simulink library "KR6_Lib"  (R2018a)
settings: Solver=VariableStepAuto  StartTime=0.0  StopTime=10.0  RelTol=1e-3
settings Model: Creator=Pedro Ramalho  LastModifiedBy=Pedro Ramalho

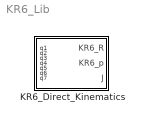
== system KR6_Lib ==
  KR6_Direct_Kinematics : MATLAB Function  TreatAsAtomicUnit=on

== matlab function KR6_Lib/KR6_Direct_Kinematics ==
  data: q1 input; KR6_R output; q2 input; q3 input; q4 input; q5 input; q6 input; q7 input; KR6_p output; J output
function [KR6_R,KR6_p,J] = KR6_Direct_Kinematics(q1,q2,q3,q4,q5,q6,q7)
%#codegen

%    This function was generated by the Symbolic Math Toolbox version 8.1.
%    09-Apr-2020 23:52:27

t2 = cos(q2);
t3 = sin(q2);
t4 = sin(q5);
t5 = cos(q5);
t6 = cos(q3);
t7 = cos(q4);
t8 = sin(q3);
t9 = sin(q4);
t13 = t2.*t6.*t7;
t14 = t2.*t8.*t9;
t10 = t13-t14;
t11 = cos(q7);
t12 = t3.*t5;
t73 = t4.*t10;
t15 = t12-t73;
t16 = sin(q7);
t17 = cos(q6);
t18 = t3.*t4;
t19 = t5.*t10;
t20 = t18+t19;
t21 = sin(q6);
t22 = t2.*t6.*t9;
t23 = t2.*t7.*t8;
t24 = t22+t23;
t25 = t17.*t20-t21.*t24;
t26 = q3+q4;
t27 = sin(t26);
t28 = cos(t26);
t29 = t21.*t28;
t30 = t5.*t17.*t27;
t31 = t29+t30;
t32 = t3.*t6.*t7;
t35 = t3.*t8.*t9;
t33 = t32-t35;
t34 = t2.*t5;
t36 = t4.*t33;
t37 = t34+t36;
t38 = t2.*t4;
t46 = t5.*t33;
t39 = t38-t46;
t40 = t17.*t39;
t41 = t3.*t6.*t9;
t42 = t3.*t7.*t8;
t43 = t41+t42;
t44 = t21.*t43;
t45 = t40+t44;
t47 = t3.*t8.*t9.*(7.0./2.0e2);
t48 = t3.*t17.*t27.*(2.0./2.5e1);
t49 = t3.*t6.*t9.*(7.3e1./2.0e2);
t50 = t3.*t7.*t8.*(7.3e1./2.0e2);
t51 = t3.*t5.*t6.*t7.*t21.*(2.0./2.5e1);
t52 = t28.*(7.3e1./2.0e2);
t53 = t27.*(7.0./2.0e2);
t54 = t8.*(6.3e1./2.0e2);
t55 = q5-q6;
t56 = sin(t55);
t57 = t27.*t56.*(1.0./2.5e1);
t58 = q5+q6;
t59 = sin(t58);
t60 = t17.*t28.*(2.0./2.5e1);
t68 = t27.*t59.*(1.0./2.5e1);
t61 = t52+t53+t54+t57+t60-t68;
t62 = t6.*t7.*(7.0./2.0e2);
t63 = t5.*t8.*t9.*t21.*(2.0./2.5e1);
t64 = t2.*(1.0./4.0e1);
t65 = t2.*t6.*(6.3e1./2.0e2);
t66 = t2.*t6.*t7.*(7.0./2.0e2);
t67 = t2.*t5.*t8.*t9.*t21.*(2.0./2.5e1);
t69 = t28.*7.3e1;
t70 = t27.*7.0;
t71 = t17.*t28.*1.6e1;
t72 = t69+t70+t71-t5.*t21.*t27.*1.6e1;
t74 = t17.*t28;
t75 = t17.*t43;
KR6_R = reshape([t15.*t16+t11.*t25,t11.*t31-t4.*t16.*t27,t16.*t37+t11.*t45,-t11.*t15+t16.*t25,t16.*t31+t4.*t11.*t27,-t11.*t37+t16.*t45,-t17.*t24-t20.*t21,t74-t5.*t21.*t27,t75-t21.*t39],[3,3]);
if nargout > 1
    KR6_p = [t64+t65+t66+t67-t2.*t6.*t9.*(7.3e1./2.0e2)-t2.*t7.*t8.*(7.3e1./2.0e2)-t2.*t8.*t9.*(7.0./2.0e2)-t3.*t4.*t21.*(2.0./2.5e1)-t2.*t17.*t27.*(2.0./2.5e1)-t2.*t5.*t6.*t7.*t21.*(2.0./2.5e1);t61;q1-t3.*(1.0./4.0e1)+t47+t48+t49+t50+t51-t3.*t6.*(6.3e1./2.0e2)-t3.*t6.*t7.*(7.0./2.0e2)-t2.*t4.*t21.*(2.0./2.5e1)-t3.*t5.*t8.*t9.*t21.*(2.0./2.5e1)];
end
if nargout > 2
    J = reshape([0.0,0.0,1.0,0.0,0.0,0.0,t3.*(-1.0./4.0e1)+t47+t48+t49+t50+t51-t3.*t6.*(6.3e1./2.0e2)-t3.*t6.*t7.*(7.0./2.0e2)-t2.*t4.*t21.*(2.0./2.5e1)-t3.*t5.*t8.*t9.*t21.*(2.0./2.5e1),0.0,-t64-t65-t66-t67+t2.*t6.*t9.*(7.3e1./2.0e2)+t2.*t7.*t8.*(7.3e1./2.0e2)+t2.*t8.*t9.*(7.0./2.0e2)+t3.*t4.*t21.*(2.0./2.5e1)+t2.*t17.*t27.*(2.0./2.5e1)+t2.*t5.*t6.*t7.*t21.*(2.0./2.5e1),0.0,1.0,0.0,-t2.*t61,t6.*(6.3e1./2.0e2)+t62+t63-t6.*t9.*(7.3e1./2.0e2)-t7.*t8.*(7.3e1./2.0e2)-t8.*t9.*(7.0./2.0e2)-t6.*t9.*t17.*(2.0./2.5e1)-t7.*t8.*t17.*(2.0./2.5e1)-t5.*t6.*t7.*t21.*(2.0./2.5e1),t3.*t61,t3,0.0,t2,t2.*t72.*(-1.0./2.0e2),t62+t63-t6.*t9.*(7.3e1./2.0e2)-t7.*t8.*(7.3e1./2.0e2)-t8.*t9.*(7.0./2.0e2)-t6.*t9.*t17.*(2.0./2.5e1)-t7.*t8.*t17.*(2.0./2.5e1)-t5.*t6.*t7.*t21.*(2.0./2.5e1),t3.*t72.*(1.0./2.0e2),t3,0.0,t2,t21.*(t12-t2.*t4.*t6.*t7+t2.*t4.*t8.*t9).*(-2.0./2.5e1),t4.*t21.*t27.*(2.0./2.5e1),t21.*(t34+t3.*t4.*t6.*t7-t3.*t4.*t8.*t9).*(-2.0./2.5e1),t2.*t27,-t28,-t3.*t27,t3.*t4.*t17.*(-2.0./2.5e1)+t2.*t6.*t9.*t21.*(2.0./2.5e1)+t2.*t7.*t8.*t21.*(2.0./2.5e1)-t2.*t5.*t6.*t7.*t17.*(2.0./2.5e1)+t2.*t5.*t8.*t9.*t17.*(2.0./2.5e1),t6.*t7.*t21.*(-2.0./2.5e1)+t8.*t9.*t21.*(2.0./2.5e1)-t5.*t6.*t9.*t17.*(2.0./2.5e1)-t5.*t7.*t8.*t17.*(2.0./2.5e1),t2.*t4.*t17.*(-2.0./2.5e1)-t3.*t6.*t9.*t21.*(2.0./2.5e1)-t3.*t7.*t8.*t21.*(2.0./2.5e1)+t3.*t5.*t6.*t7.*t17.*(2.0./2.5e1)-t3.*t5.*t8.*t9.*t17.*(2.0./2.5e1),t15,-t4.*t27,t34+t4.*(t32-t35),0.0,0.0,0.0,t17.*t24+t20.*t21,-t74+t5.*t21.*t27,-t75+t21.*t39],[6,7]);
end
